simulink model "SystemeComplet"  (R2019b)
settings: Solver=VariableStepAuto  StartTime=0.0  StopTime=10  RelTol=1e-3
libraries: dspsrcs4 x2
settings Model: Creator=jeanz  LastModifiedBy=jeanz

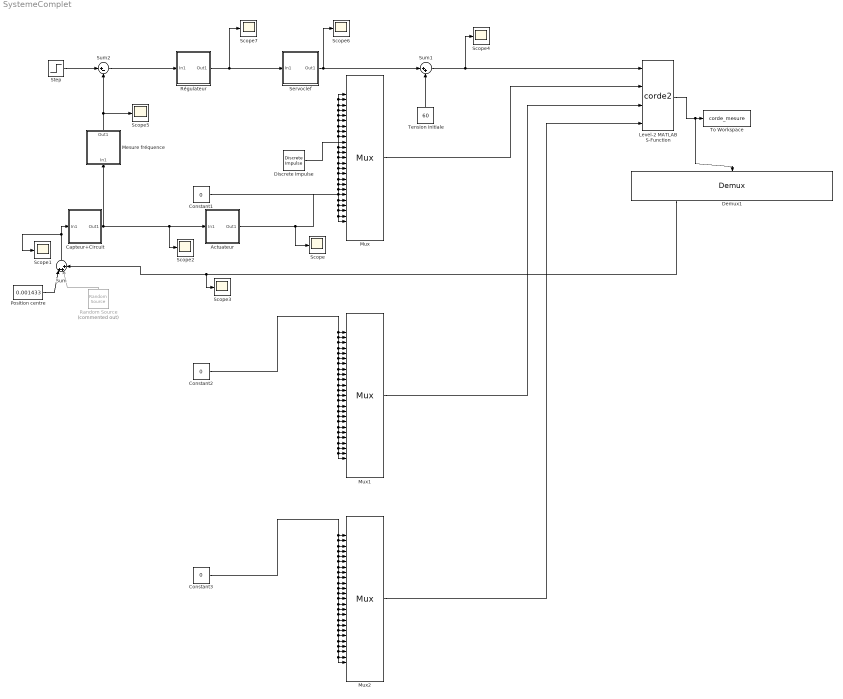
== system SystemeComplet ==
  Actuateur : Subsystem
  Capteur+Circuit : Subsystem
  Constant1 : Constant  Value=0
  Constant2 : Constant  Value=0
  Constant3 : Constant  Value=0
  Demux1 : Demux  Outputs=25
  Discrete Impulse : dspsrcs4/Discrete  Impulse  Delay=0  SampleTime=1  FrameSample=1  OutputFrames=off  dataType=double  isSigned=on  wordLen=16  udDataType=sfix(16)  fracBitsMode=Best precision  numFracBits=15  OutDataTypeStr=double  LastOutDataTypeStr=double
  Level-2 MATLAB S-Function : M-S-Function  FunctionName=corde2  Parameters=0.00325, 0.44, 0.0326, 25
  Mesure fréquence : Subsystem
  Mux : Mux  Inputs=25
  Mux1 : Mux  Inputs=25
  Mux2 : Mux  Inputs=25
  Position centre : Constant  Value=0.001433
  Random Source : dspsrcs4/Random Source  Commented=on  SrcType=Uniform  NormMethod=Ziggurat  CltLength=12  MinVal=-0.0001  MaxVal=0.0001  MeanVal=0  VarVal=1  RepMode=Not repeatable  rawSeed=1  IsInherit=off  SampMode=Discrete  SampTime=1  SampFrame=1  DataType=Double  OutComplex=Real  OutputFrames=off
  Régulateur : Subsystem
  Scope{,1..7} (8 alike) : Scope
  Servoclef : Subsystem
  Step : Step  Time=4  Before=200  After=220  SampleTime=0
  Sum : Sum  Inputs=|+++
  Sum1 : Sum  Inputs=|++
  Sum2 : Sum  Inputs=|+-
  Tension initiale : Constant  Value=60
  To Workspace : ToWorkspace  VariableName=corde_mesure  SaveFormat=Timeseries  SampleTime=0.0005
  wires:
  Mux2/1 -> Level-2 MATLAB S-Function/4
  Constant2/1 -> Mux1/1, Mux1/2, Mux1/3, Mux1/4, Mux1/6, Mux1/12, Mux1/20, Mux1/25, Mux1/24, Mux1/23, Mux1/22, Mux1/21, Mux1/19, Mux1/18, Mux1/17, Mux1/16, Mux1/15, Mux1/14, Mux1/13, Mux1/11, Mux1/10, Mux1/9, Mux1/8, Mux1/7, Mux1/5
  Constant3/1 -> Mux2/1, Mux2/2, Mux2/3, Mux2/4, Mux2/6, Mux2/25, Mux2/24, Mux2/23, Mux2/22, Mux2/21, Mux2/20, Mux2/19, Mux2/18, Mux2/17, Mux2/16, Mux2/15, Mux2/14, Mux2/13, Mux2/12, Mux2/11, Mux2/10, Mux2/9, Mux2/8, Mux2/7, Mux2/5
  Mux/1 -> Level-2 MATLAB S-Function/2
  Mux1/1 -> Level-2 MATLAB S-Function/3
  Constant1/1 -> Mux/16, Mux/15, Mux/14, Mux/13, Mux/12, Mux/11, Mux/9, Mux/8, Mux/7, Mux/6, Mux/5, Mux/4, Mux/3, Mux/1, Mux/2, Mux/17, Mux/18, Mux/19, Mux/25, Mux/24, Mux/23, Mux/22, Mux/21
  Level-2 MATLAB S-Function/1 -> Demux1/1, To Workspace/1
  Actuateur/1(Out1) -> Scope/1, Mux/20
  Capteur+Circuit/1(Out1) -> Mesure fréquence/1(In1), Scope2/1, Actuateur/1(In1)
  Mesure fréquence/1(Out1) -> Sum2/2, Scope5/1
  Sum/1 -> Scope1/1, Capteur+Circuit/1(In1)
  Demux1/6 -> Sum/3, Scope3/1
  Position centre/1 -> Sum/1
  Tension initiale/1 -> Sum1/2
  Servoclef/1(Out1) -> Sum1/1, Scope6/1
  Sum1/1 -> Level-2 MATLAB S-Function/1, Scope4/1
  Random Source/1 -> Sum/2
  Discrete Impulse/1 -> Mux/10
  Step/1 -> Sum2/1
  Régulateur/1(Out1) -> Scope7/1, Servoclef/1(In1)
  Sum2/1 -> Régulateur/1(In1)

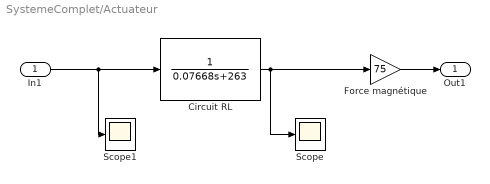
== system SystemeComplet/Actuateur ==
  In1 : Inport
  Circuit RL : TransferFcn  Denominator=[0.07668 263]
  Force magnétique : Gain  Gain=75
  Scope : Scope
  Scope1 : Scope
  Out1 : Outport
  wires:
  Force magnétique/1 -> Out1/1
  Circuit RL/1 -> Force magnétique/1, Scope/1
  In1/1 -> Scope1/1, Circuit RL/1

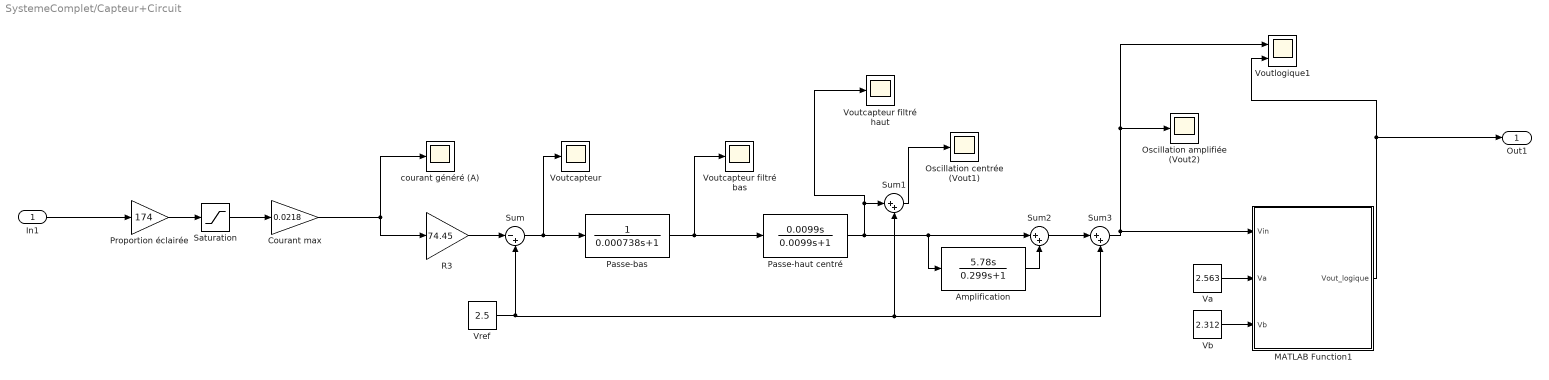
== system SystemeComplet/Capteur+Circuit ==
  In1 : Inport
  "Amplification " : TransferFcn  Numerator=[5.78 0]  Denominator=[0.299 1]
  Courant max : Gain  Gain=0.0218
  MATLAB Function1 : MATLAB Function  TreatAsAtomicUnit=on
  "Oscillation amplifiée (Vout2) " : Scope
  Oscillation centrée (Vout1) : Scope
  Passe-bas : TransferFcn  Denominator=[0.000738 1]
  "Passe-haut centré " : TransferFcn  Numerator=[0.0099 0]  Denominator=[0.0099 1]
  Proportion éclairée : Gain  Gain=174
  R3 : Gain  Gain=74.45
  Saturation : Saturate  UpperLimit=0.497  LowerLimit=0
  Sum : Sum  Inputs=|-+
  Sum1 : Sum  Inputs=|++
  Sum2 : Sum  Inputs=|++
  Sum3 : Sum  Inputs=|++
  "Va " : Constant  Value=2.563
  Vb : Constant  Value=2.312
  "Voutcapteur " : Scope
  Voutcapteur filtré bas : Scope
  Voutcapteur filtré haut : Scope
  Voutlogique1 : Scope  NumInputPorts=2
  "Vref " : Constant  Value=2.5
  "courant généré (A) " : Scope
  Out1 : Outport
  wires:
  "Amplification "/1 -> Sum2/2
  Sum3/1 -> Voutlogique1/1, "Oscillation amplifiée (Vout2) "/1, MATLAB Function1/1(Vin)
  "Vref "/1 -> Sum/2, Sum3/2, Sum1/2
  Sum/1 -> "Voutcapteur "/1, Passe-bas/1
  R3/1 -> Sum/1
  "Passe-haut centré "/1 -> Sum2/1, "Amplification "/1, Voutcapteur filtré haut/1, Sum1/1
  Vb/1 -> MATLAB Function1/3(Vb)
  Passe-bas/1 -> Voutcapteur filtré bas/1, "Passe-haut centré "/1
  Sum2/1 -> Sum3/1
  Sum1/1 -> Oscillation centrée (Vout1)/1
  MATLAB Function1/1(Vout_logique) -> Out1/1, Voutlogique1/2
  "Va "/1 -> MATLAB Function1/2(Va)
  Saturation/1 -> Courant max/1
  Proportion éclairée/1 -> Saturation/1
  Courant max/1 -> R3/1, "courant généré (A) "/1
  In1/1 -> Proportion éclairée/1

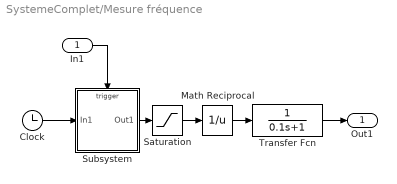
== system SystemeComplet/Mesure fréquence ==
  In1 : Inport
  Clock : Clock
  Math Reciprocal : Math  Operator=reciprocal  SaturateOnIntegerOverflow=on
  Saturation : Saturate  UpperLimit=1  LowerLimit=0.001
  Subsystem : Subsystem
  Transfer Fcn : TransferFcn  Denominator=[0.1 1]
  Out1 : Outport
  wires:
  In1/1 -> Subsystem/Trigger
  Clock/1 -> Subsystem/1(In1)
  Subsystem/1(Out1) -> Saturation/1
  Saturation/1 -> Math Reciprocal/1
  Math Reciprocal/1 -> Transfer Fcn/1
  Transfer Fcn/1 -> Out1/1

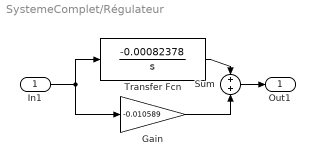
== system SystemeComplet/Régulateur ==
  In1 : Inport
  Gain : Gain  Gain=-0.010589
  Sum : Sum  Inputs=+|+
  Transfer Fcn : TransferFcn  Numerator=[-0.00082378]  Denominator=[1 0]
  Out1 : Outport
  wires:
  In1/1 -> Gain/1, Transfer Fcn/1
  Sum/1 -> Out1/1
  Transfer Fcn/1 -> Sum/1
  Gain/1 -> Sum/2

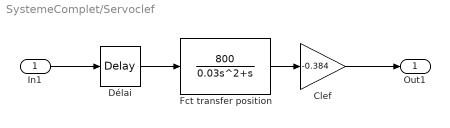
== system SystemeComplet/Servoclef ==
  In1 : Inport
  Clef : Gain  Gain=-0.384
  Délai : TransportDelay  DelayTime=0.01
  Fct transfer position : TransferFcn  Numerator=[800]  Denominator=[0.03 1 0]
  Out1 : Outport
  wires:
  Fct transfer position/1 -> Clef/1
  Clef/1 -> Out1/1
  Délai/1 -> Fct transfer position/1
  In1/1 -> Délai/1

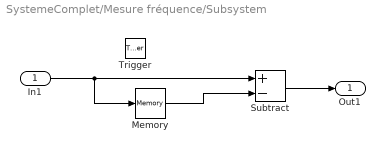
== system SystemeComplet/Mesure fréquence/Subsystem ==
  In1 : Inport
  Trigger : TriggerPort  VariantControl=Variant  PortDimensions=1
  Memory : Memory  InheritSampleTime=on
  Subtract : Sum  Inputs=+-
  Out1 : Outport
  wires:
  In1/1 -> Memory/1, Subtract/1
  Memory/1 -> Subtract/2
  Subtract/1 -> Out1/1

== matlab function SystemeComplet/Capteur+Circuit/MATLAB Function1 ==
  data: Vin input; Vout_logique output; Va input; Vb input
function Vout_logique = fcn(Vin, Va, Vb)

Vout_logique = 0;
if Vin > Va && Vout_logique == 5
    Vout_logique = 0;
end
if Vin < Vb && Vout_logique == 0
    Vout_logique = 5;
end
end
